simulink model "testing_udt"  (R2018b)
settings: Solver=FixedStepDiscrete  StartTime=0.0  StopTime=10  FixedStep=0.05  RelTol=1e-3  EnableMultiTasking=on
libraries: libudt x2, simulink x1, sldrtlib x1
settings Model: SimulationMode=external  Creator=Lenovo  LastModifiedBy=Lenovo
settings SolverCC: PositivePriorityOrder=on
settings OptimizationCC: DefaultParameterBehavior=Inlined  UseDivisionForNetSlopeComputation=on  UseFloatMulNetSlope=on  InlineInvariantSignals=on  PassReuseOutputArgsThreshold=0  EfficientFloat2IntCast=on  MaxStackSize=64  OptimizeBlockOrder=speed  DifferentSizesBufferReuse=on
settings DebuggingCC: SignalInfNanChecking=error  IntegerOverflowMsg=error  ParameterTunabilityLossMsg=error  AssertControl=DisableAll  LibraryContextMissingDiagnostic=none
settings ModelReferenceCC: ModelReferenceMinAlgLoopOccurrences=on
settings SFSimCC: SimUseLocalCustomCode=off  MATLABDynamicMemAlloc=off
settings RTWCC: SystemTargetFile=sldrt.tlc  TemplateMakefile=sldrt.tmf  Description=Simulink Desktop Real-Time  GenerateReport=on  RTWUseLocalCustomCode=off  Toolchain=GNU GCC BeagleBone Blue  BuildConfiguration=Faster Runs  RTWCompilerOptimization=on
settings CodeAppCC: ForceParamTrailComments=on  MaxIdLength=95  OperatorAnnotations=on
settings SimulinkDesktopRealTimeCC: TargetPreCompLibLocation=C:\Program Files\MATLAB\R2018b\toolbox\sldrt\lib\win64  TargetLangStandard=C89/C90 (ANSI)  PreserveStateflowLocalDataDimensions=off

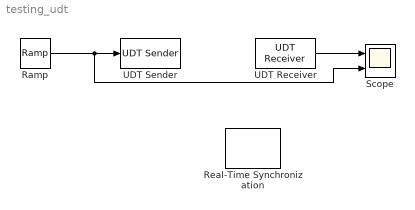
== system testing_udt ==
  Ramp : simulink/Sources/Ramp  slope=0.5  start=0  InitialOutput=0
  Real-Time Synchronization : sldrtlib/Real-Time Synchronization  SampleTime=0.05  MaxMissedTicks=10  ShowMissedTicks=off  YieldWhenWaiting=off
  Scope : Scope  NumInputPorts=2
  UDT Receiver : libudt/UDT Receiver  hostaddress='127.0.0.1'  hostport='2000'  datawidth=1  sampletime=0.05
  UDT Sender : libudt/UDT Sender  hostaddress='127.0.0.1'  hostport='2000'  sampletime=0.05
  wires:
  UDT Receiver/1 -> Scope/1
  Ramp/1 -> Scope/2, UDT Sender/1
